simulink model "Model"  (R2017b)
settings: Solver=VariableStepAuto  StartTime=0.0  StopTime=10.0  RelTol=1e-3
undefined symbols (not defined in the file): A1, A2, A3, c0, c1, c2, k, simSwitch, u1, u2, x0
settings Model: Creator=lasse  LastModifiedBy=lasse

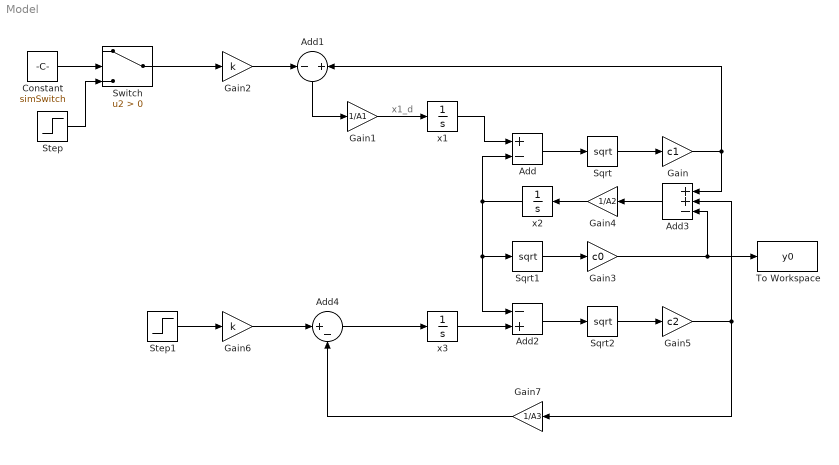
== system Model ==
  note: x1_d
  Add : Sum  Inputs=+-
  Add1 : Sum  Inputs=-+
  Add2 : Sum  Inputs=-+
  Add3 : Sum  Inputs=++-
  Add4 : Sum  Inputs=|+-
  Constant : Constant  Value=simSwitch
  Gain : Gain  Gain=c1
  Gain1 : Gain  Gain=1/A1
  Gain2 : Gain  Gain=k
  Gain3 : Gain  Gain=c0
  Gain4 : Gain  Gain=1/A2
  Gain5 : Gain  Gain=c2
  Gain6 : Gain  Gain=k
  Gain7 : Gain  Gain=1/A3
  Sqrt : Sqrt  SaturateOnIntegerOverflow=on
  Sqrt1 : Sqrt  SaturateOnIntegerOverflow=on
  Sqrt2 : Sqrt  SaturateOnIntegerOverflow=on
  Step : Step  Time=0  After=u1  SampleTime=0
  Step1 : Step  Time=0  After=u2  SampleTime=0  ZeroCross=off
  Switch : Switch  Criteria=u2 > Threshold
  To Workspace : ToWorkspace  VariableName=y0  SaveFormat=Timeseries  SampleTime=-1
  x1 : Integrator  InitialCondition=x0(1)
  x2 : Integrator  InitialCondition=x0(2)
  x3 : Integrator  InitialCondition=x0(3)
  wires:
  x1/1 -> Add/1
  x2/1 -> Add/2, Sqrt1/1, Add2/1
  Add/1 -> Sqrt/1
  Sqrt/1 -> Gain/1
  Gain1/1 -> x1/1
  Add1/1 -> Gain1/1
  Gain/1 -> Add3/1, Add1/2
  Gain2/1 -> Add1/1
  x3/1 -> Add2/2
  Sqrt1/1 -> Gain3/1
  Gain4/1 -> x2/1
  Add3/1 -> Gain4/1
  Gain3/1 -> To Workspace/1, Add3/3
  Add2/1 -> Sqrt2/1
  Sqrt2/1 -> Gain5/1
  Gain5/1 -> Gain7/1, Add3/2
  Step1/1 -> Gain6/1
  Add4/1 -> x3/1
  Gain6/1 -> Add4/1
  Gain7/1 -> Add4/2
  Step/1 -> Switch/3
  Switch/1 -> Gain2/1
  Constant/1 -> Switch/2
